simulink model "MAruti_Swift_Desire_Powerd_by_50hp_dc_Motor"  (R2023a)
settings: Solver=ode45  StartTime=0.0  StopTime=100  RelTol=1e-3  EnableMultiTasking=on
libraries: spsDCMachineLib x1, simulink x1, spsControlledVoltageSourceLib x1, spsDCVoltageSourceLib x1, spspowerguiLib x1
settings Model: Creator=INTEL  LastModifiedBy=vashe
settings SolverCC: AlgebraicLoopSolver=LineSearch
settings DataIOCC: LimitDataPoints=on  SaveFormat=Array  ReturnWorkspaceOutputs=off
settings OptimizationCC: LifeSpan=inf
settings DebuggingCC: SolverPrmCheckMsg=warning  UnconnectedInputMsg=warning  UnconnectedOutputMsg=warning  UnconnectedLineMsg=warning  SFUnexpectedBacktrackingDiag=warning  SFNoUnconditionalDefaultTransitionDiag=warning  SFExecutionAtInitializationDiag=none  ArithmeticOperatorsInVariantConditions=warning
settings HardwareCC: ProdBitPerPointer=32  ProdBitPerSizeT=32  ProdBitPerPtrDiffT=32  ProdLargestAtomicFloat=None  ProdIntDivRoundTo=Undefined  ProdEndianess=Unspecified  ProdWordSize=32  ProdHWDeviceType=32-bit Generic
settings ModelReferenceCC: PropagateSignalLabelsOutOfModel=off
settings SFSimCC: SimUseLocalCustomCode=off  CustomCodeUndefinedFunction=UseInterfaceOnly
settings RTWCC: RTWUseLocalCustomCode=off
settings CodeAppCC: StateflowObjectComments=on
settings GRTTargetCC: TargetLangStandard=C89/C90 (ANSI)
settings ConfigComp: CovMetricSettings=dw  CovSaveCumulativeToWorkspaceVar=on  CovSaveSingleToWorkspaceVar=on  CovExternalEMLEnable=off  CovSFcnEnable=off
settings SimscapeCC: SimscapeNormalizeSystem=off

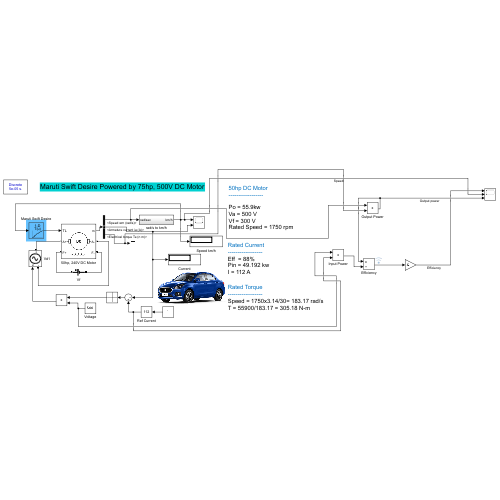
[thumbnail: Simulink's stored preview of the top-level diagram]
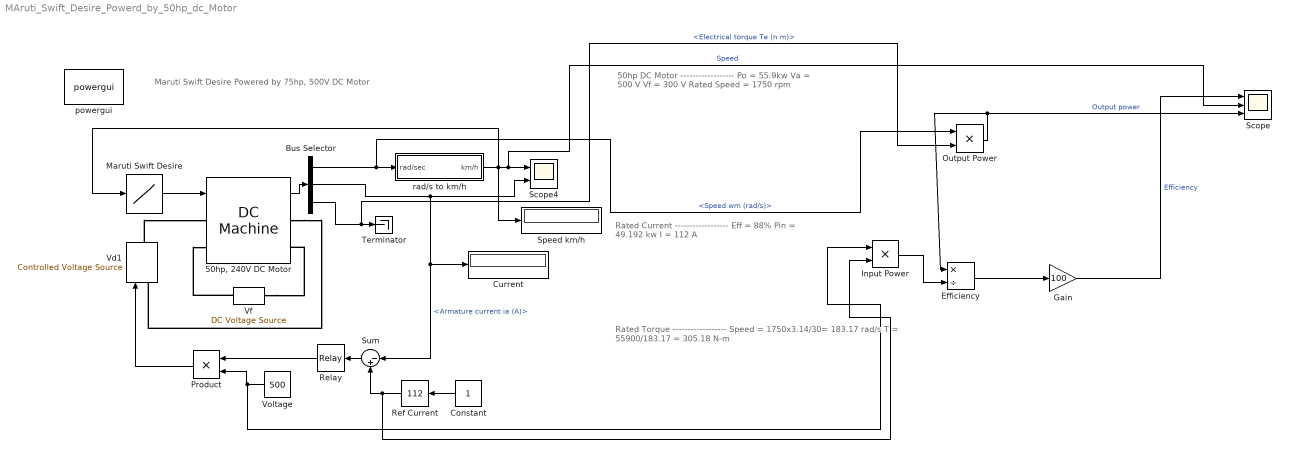
== system MAruti_Swift_Desire_Powerd_by_50hp_dc_Motor ==
  note: Maruti Swift Desire Powered by 75hp, 500V DC Motor
  note: 50hp DC Motor
      | ------------------
      |
      | Po = 55.9kw
      | Va = 500 V
      | Vf = 300 V
      | Rated Speed = 1750 rpm
  note: Rated Current
      | ------------------
      | Eff = 88%
      | Pin = 49.192 kw
      | I = 112 A
  note: Rated Torque
      | ------------------
      | Speed = 1750x3.14/30= 183.17 rad/s
      | T = 55900/183.17 = 305.18 N-m
  "50hp, 240V DC Motor" : spsDCMachineLib/DC Machine  PresetModel=No  MechanicalLoad=Torque TL  FieldType=Wound  ShowDetailedParameters=on  MeasurementBus=off  RLa=[0.2828 0.004453]  RLf=[69.77 9.413]  Laf=0.5899  MachineConstant=Torque constant (N.m/A)  Ke=1.8  Kt=1.8  J=103.92  Bm=0.009298  Tf=7.929  w0=1  Ifinit=4.29984233911423  TsPowergui=0  TsBlock=-1
  Bus Selector : BusSelector  OutputSignals=Speed wm (rad/s),Armature current ia (A),Electrical torque Te (n m)
  Constant : Constant
  Current : Display
  Efficiency : Product  Inputs=*/
  Gain : Gain  Gain=100
  Input Power : Product
  Maruti Swift Desire : Lookup_n-D  NumberOfTableDimensions=1  BreakpointsForDimension1=[0, 50, 60, 70, 80, 100, 150, 200, 250, 300, 350]  Table=[0,20.37,27.76, 34.83, 41.62, 54.38, 82.49, 106.4, 127.2,145.7,162.4]  InternalRulePriority=Speed  RndMeth=Simplest
  Output Power : Product
  Product : Product
  Ref Current : simulink/Math Operations/Slider Gain  gain=112  low=0  high=187
  Relay : Relay  OnSwitchValue=2  OffSwitchValue=-2
  Scope : Scope  NumInputPorts=3
  Scope4 : Scope  NumInputPorts=2
  Speed km/h : Display
  Sum : Sum  Inputs=|-+
  Terminator : Terminator
  Vd1 : spsControlledVoltageSourceLib/Controlled Voltage Source  Initialize=on  Source_Type=DC  Amplitude=0  Phase=0  Frequency=0  Measurements=None
  Vf : spsDCVoltageSourceLib/DC Voltage Source  Amplitude=300  Measurements=None
  Voltage : Constant  Value=500
  powergui : spspowerguiLib/powergui  Priority=1  SimulationMode=Discrete  SampleTime=50e-6  frequency=60  Iterations=50  frequencyindice=0  Pbase=100e6  ErrMax=1e-4  UnitsV=kV  UnitsW=MW  buscounter=0  FunctionMessages=off  echomessages=off  EnableUseOfTLC=off  CurrentSourceSwitches=off  DisableSnubberDevices=off  DisableRonSwitches=off  DisableVfSwitches=off  DisplayEquations=off  AutomaticDiscreteSolvers=off  SolverType=Tustin/Backward Euler (TBE)  Interpol=off  ExternalGateDelay=off  methode=off  Ts=100  x0status=blocks  SPID=off  SwTol=0  HookPort=off  NonlinearTolerance=1e-4  nMaxIteration=100  ContinueOnMaxIteration=off  RestoreLinks=warning  ResistiveCurrentMeasurement=off  Frange=[0:2:500]  Ylog=off  Xlog=on  ShowGrid=off  save=off  variable=ZData  structure=0  ZoomFFT=off  StartTime=0.0  cycles=1  DisplayStyle=1  fundamental=60  FreqAxis=off  MaxFrequency=1000  frequencyindicesteady=1  RmsSteady=1  display=off
  rad/s to km/h : Subsystem
  wires:
  Maruti Swift Desire/1 -> "50hp, 240V DC Motor"/1
  "50hp, 240V DC Motor"/1 -> Bus Selector/1
  rad/s to km/h/1(km/h) -> Speed km/h/1, Scope/2, Scope4/1, Maruti Swift Desire/1  "Speed"
  Bus Selector/1 -> Output Power/1, rad/s to km/h/1(rad/sec)  "<Speed wm (rad/s)>"
  Bus Selector/3 -> Output Power/2, Terminator/1  "<Electrical torque Te (n m)>"
  Bus Selector/2 -> Sum/1, Current/1, Scope4/2  "<Armature current ia (A)>"
  Constant/1 -> Ref Current/1
  Sum/1 -> Relay/1
  Relay/1 -> Product/1
  Voltage/1 -> Input Power/1, Product/2
  Product/1 -> Vd1/1
  Ref Current/1 -> Input Power/2, Sum/2
  Output Power/1 -> Efficiency/1, Scope/3  "Output power"
  Input Power/1 -> Efficiency/2
  Efficiency/1 -> Gain/1
  Gain/1 -> Scope/1  "Efficiency"
  connections:
  Vf/RConn1 -- "50hp, 240V DC Motor"/LConn2
  Vf/LConn1 -- "50hp, 240V DC Motor"/RConn2
  Vd1/RConn1 -- "50hp, 240V DC Motor"/LConn1
  "50hp, 240V DC Motor"/RConn1 -- Vd1/LConn1

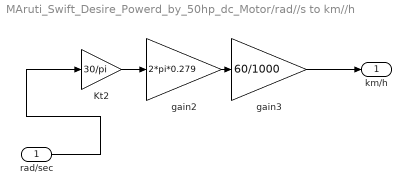
== system MAruti_Swift_Desire_Powerd_by_50hp_dc_Motor/rad//s to km//h ==
  rad/sec : Inport
  Kt2 : Gain  Gain=30/pi
  gain2 : Gain  Gain=2*pi*0.279
  gain3 : Gain  Gain=60/1000
  km/h : Outport
  wires:
  Kt2/1 -> gain2/1
  gain2/1 -> gain3/1
  gain3/1 -> km/h/1
  rad/sec/1 -> Kt2/1
